simulink subsystem "Sensores"  (R2026a)
settings: Solver=VariableStepAuto
settings Model: Creator=admin  LastModifiedBy=admin

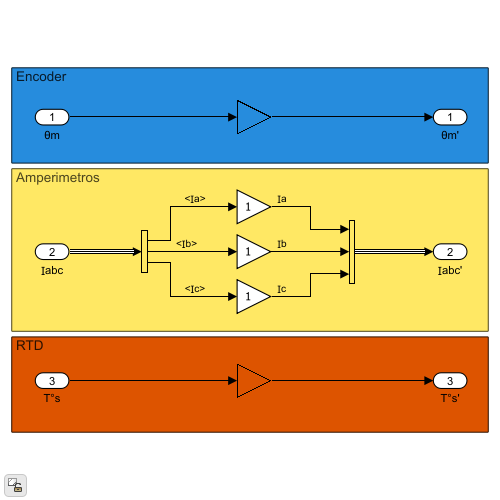
[thumbnail: Simulink's stored preview of the top-level diagram]
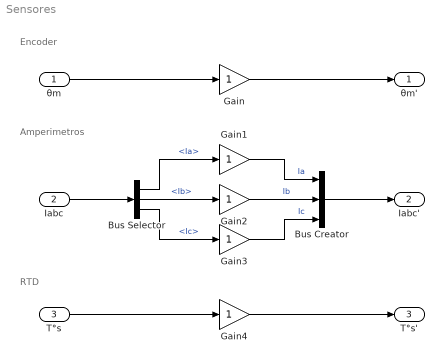
== system Sensores ==
  note: Encoder
  note: Amperimetros
  note: RTD
  θm : Inport
  Ⅰabc : Inport  Port=2
  T°s : Inport  Port=3
  Bus Creator : BusCreator  Inputs=3
  Bus Selector : BusSelector  OutputSignals=Ⅰa,Ⅰb,Ⅰc
  Gain{,1..4} (5 alike) : Gain
  θm' : Outport
  Ⅰabc' : Outport  Port=2
  T°s' : Outport  Port=3
  wires:
  θm/1 -> Gain/1
  Gain/1 -> θm'/1
  T°s/1 -> Gain4/1
  Gain4/1 -> T°s'/1
  Bus Creator/1 -> Ⅰabc'/1
  Ⅰabc/1 -> Bus Selector/1
  Bus Selector/1 -> Gain1/1  "<Ⅰa>"
  Bus Selector/2 -> Gain2/1  "<Ⅰb>"
  Bus Selector/3 -> Gain3/1  "<Ⅰc>"
  Gain2/1 -> Bus Creator/2  "Ⅰb"
  Gain1/1 -> Bus Creator/1  "Ⅰa"
  Gain3/1 -> Bus Creator/3  "Ⅰc"
